simulink model "firmware"  (R2020a)
settings: Solver=FixedStepAuto  StartTime=0.0  StopTime=50.0  FixedStep=1e-3  RelTol=1e-3  EnableMultiTasking=on
undefined symbols (not defined in the file): A0, A1, A3, D0, D1, D10, D11, D12, D13, D2, D3, D4, D5, D6, D7, D8, D9, PTA0, PTA1, PTA2, PTB11, PTB2, PTB23, PTB3, PTB9, PTC16, PTC17, PTC2, PTC3, PTC4, PTD0, PTD1, PTD2, PTD3
libraries: etargetslib x44, frdmk64flib x22, dspstat3 x1
(part 2 of 2)

== system firmware/1.1.2 InputProcessing/1.1.2.4 CalculateUnsensedPace ==
  note: This block sets the LRL as a pulse period, later
      | used by AOO and VOO
  LowerRateLimit : Inport
  Data Type Conversion1 : DataTypeConversion  OutDataTypeStr=single
  Fcn2 : Fcn  Expr=u/60000
  Math Function1 : Math  Operator=reciprocal  SaturateOnIntegerOverflow=on
  f_aooInterval : Outport
  f_vooInterval : Outport  Port=2
  wires:
  Math Function1/1 -> f_vooInterval/1, f_aooInterval/1
  Data Type Conversion1/1 -> Fcn2/1
  Fcn2/1 -> Math Function1/1
  LowerRateLimit/1 -> Data Type Conversion1/1

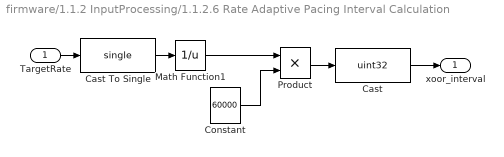
== system firmware/1.1.2 InputProcessing/1.1.2.6 Rate Adaptive Pacing Interval Calculation ==
  TargetRate : Inport  OutDataTypeStr=single
  Cast : DataTypeConversion  OutDataTypeStr=uint32
  Cast To Single : DataTypeConversion  OutDataTypeStr=single
  Constant : Constant  Value=60000
  Math Function1 : Math  Operator=reciprocal  SaturateOnIntegerOverflow=on
  Product : Product
  xoor_interval : Outport  OutDataTypeStr=uint32
  wires:
  Constant/1 -> Product/2
  Math Function1/1 -> Product/1
  Product/1 -> Cast/1
  Cast/1 -> xoor_interval/1
  TargetRate/1 -> Cast To Single/1
  Cast To Single/1 -> Math Function1/1

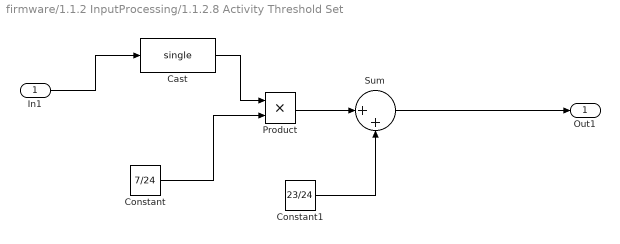
== system firmware/1.1.2 InputProcessing/1.1.2.8 Activity Threshold Set  ==
  In1 : Inport
  Cast : DataTypeConversion  OutDataTypeStr=single
  Constant : Constant  Value=7/24
  Constant1 : Constant  Value=23/24
  Product : Product
  Sum : Sum  Inputs=|++
  Out1 : Outport
  wires:
  Constant/1 -> Product/2
  Constant1/1 -> Sum/2
  Product/1 -> Sum/1
  Sum/1 -> Out1/1
  In1/1 -> Cast/1
  Cast/1 -> Product/1

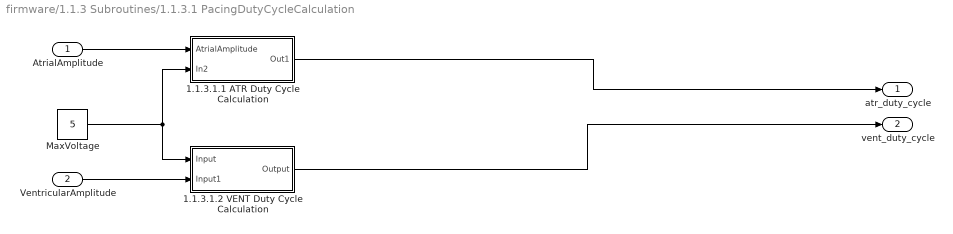
== system firmware/1.1.3 Subroutines/1.1.3.1 PacingDutyCycleCalculation ==
  AtrialAmplitude : Inport
  VentricularAmplitude : Inport  Port=2
  1.1.3.1.1 ATR Duty Cycle Calculation : Subsystem
  1.1.3.1.2 VENT Duty Cycle Calculation : Subsystem
  MaxVoltage : Constant  Value=5
  atr_duty_cycle : Outport
  vent_duty_cycle : Outport  Port=2
  wires:
  MaxVoltage/1 -> 1.1.3.1.2 VENT Duty Cycle Calculation/1(Input), 1.1.3.1.1 ATR Duty Cycle Calculation/2(In2)
  AtrialAmplitude/1 -> 1.1.3.1.1 ATR Duty Cycle Calculation/1(AtrialAmplitude)
  VentricularAmplitude/1 -> 1.1.3.1.2 VENT Duty Cycle Calculation/2(Input1)
  1.1.3.1.1 ATR Duty Cycle Calculation/1(Out1) -> atr_duty_cycle/1
  1.1.3.1.2 VENT Duty Cycle Calculation/1(Output) -> vent_duty_cycle/1

== system firmware/1.1.3 Subroutines/HIGH_or_LOW ==
  HIGH : Constant  Value=true
  LOW : Constant  Value=false
  Output : Outport
  Output1 : Outport  Port=2
  wires:
  LOW/1 -> Output1/1
  HIGH/1 -> Output/1

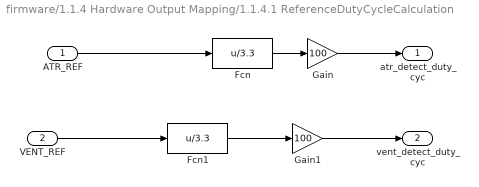
== system firmware/1.1.4 Hardware Output Mapping/1.1.4.1 ReferenceDutyCycleCalculation ==
  ATR_REF : Inport
  VENT_REF : Inport  Port=2
  Fcn : Fcn  Expr=u/3.3
  Fcn1 : Fcn  Expr=u/3.3
  Gain : Gain  Gain=100
  Gain1 : Gain  Gain=100
  atr_detect_duty_cyc : Outport
  vent_detect_duty_cyc : Outport  Port=2
  wires:
  Fcn/1 -> Gain/1
  VENT_REF/1 -> Fcn1/1
  Gain/1 -> atr_detect_duty_cyc/1
  Fcn1/1 -> Gain1/1
  Gain1/1 -> vent_detect_duty_cyc/1
  ATR_REF/1 -> Fcn/1

== system firmware/1.1.4 Hardware Output Mapping/1.1.4.2 Ventricular Pacing Inhibit ==
  VENT_CMP_REF_PWM : Inport
  VentPaceInhibit : Inport  Port=2
  Constant : Constant  Value=0
  Switch : Switch  Criteria=u2 > Threshold  Threshold=0.5
  Out1 : Outport
  wires:
  VENT_CMP_REF_PWM/1 -> Switch/3
  Constant/1 -> Switch/1
  VentPaceInhibit/1 -> Switch/2
  Switch/1 -> Out1/1

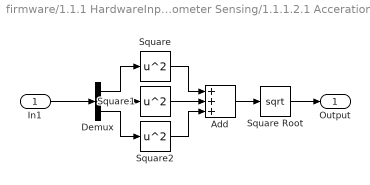
== system firmware/1.1.1 HardwareInputMapping/1.1.1.2 Accelerometer Sensing/1.1.1.2.1 Acceration Magnitude Calculation ==
  In1 : Inport
  Add : Sum  Inputs=+++
  Demux : Demux  Outputs=3
  Square : Math  Operator=square  SaturateOnIntegerOverflow=on
  Square Root : Sqrt  SaturateOnIntegerOverflow=on
  Square1 : Math  Operator=square  SaturateOnIntegerOverflow=on
  Square2 : Math  Operator=square  SaturateOnIntegerOverflow=on
  Output : Outport
  wires:
  Demux/1 -> Square/1
  Demux/2 -> Square1/1
  Demux/3 -> Square2/1
  Square/1 -> Add/1
  Square1/1 -> Add/2
  Square2/1 -> Add/3
  Add/1 -> Square Root/1
  Square Root/1 -> Output/1
  In1/1 -> Demux/1

== system firmware/1.1.3 Subroutines/1.1.3.1 PacingDutyCycleCalculation/1.1.3.1.1 ATR Duty Cycle Calculation ==
  AtrialAmplitude : Inport
  In2 : Inport  Port=2
  % : Constant  Value=100
  Divide : Product  Inputs=*/
  Product : Product
  Out1 : Outport
  wires:
  Divide/1 -> Product/1
  %/1 -> Product/2
  AtrialAmplitude/1 -> Divide/1
  In2/1 -> Divide/2
  Product/1 -> Out1/1

== system firmware/1.1.3 Subroutines/1.1.3.1 PacingDutyCycleCalculation/1.1.3.1.2 VENT Duty Cycle Calculation ==
  Input : Inport
  Input1 : Inport  Port=2
  % : Constant  Value=100
  Divide : Product  Inputs=*/
  Product : Product
  Output : Outport
  wires:
  Input/1 -> Divide/2
  Input1/1 -> Divide/1
  %/1 -> Product/2
  Divide/1 -> Product/1
  Product/1 -> Output/1

== stateflow chart firmware/1.1.2 InputProcessing/1.1.2.3 WatchdogTimerForPulseDetection ==
  state HysterisisSelection
    entry:
    time_minute = 60000; % ms/s
    smoothing_rate= InstHeartRate*(1-rs_down);
    total_lower_rate_time = 0;
  state DDDR
    entry:
    during:
    %tot_wait_time = time_minute-((ARP+AtrialPulseWidth)*smoothing_rate);
    %wait_time = tot_wait_time / smoothing_rate;
    total_XXIR_rate_time = time_minute-((p_v_a_r_p+AV_delay+AtrialPulseWidth)*XXIR_PPM);
    wait_time_XXIR= total_XXIR_rate_time/ XXIR_PPM;
    %For LRL so might not need for this mode, but again, left it here for now
    total_lower_rate_time = time_minute-((ARP+AtrialPulseWidth)*LRL);
    wait_time_LRL= total_lower_rate_time/ LRL;
    %For hysterisis so might not be needed for AAIR, but doesn't hurt to leave for now
    total_lower_rate_time_hys= time_minute - ((ARP + AtrialPulseWidth)*HRL);
    wait_time_LRL_hys= total_lower_rate_time_hys/ HRL;
  state AAI
    entry:
    tot_wait_time = time_minute-((ARP+AtrialPulseWidth)*smoothing_rate);
    wait_time = tot_wait_time / smoothing_rate;
    total_lower_rate_time = time_minute-((ARP+AtrialPulseWidth)*LRL);
    %total_lower_rate_time = time_minute - ((250 + 0.4)*50);
    wait_time_LRL= total_lower_rate_time/ LRL;
    %total_lower_rate_time_hys= time_minute - ((250 + 0.4)*45);
    %wait_time_LRL_hys= total_lower_rate_time_hys/ 45;
    total_lower_rate_time_hys= time_minute - ((ARP + AtrialPulseWidth)*HRL);
    wait_time_LRL_hys= total_lower_rate_time_hys/ HRL;
  state AAIR
    entry:
    during:
    %tot_wait_time = time_minute-((ARP+AtrialPulseWidth)*smoothing_rate);
    %wait_time = tot_wait_time / smoothing_rate;
    total_XXIR_rate_time = time_minute-((ARP+AtrialPulseWidth)*XXIR_PPM);
    wait_time_XXIR= total_XXIR_rate_time/ XXIR_PPM;
    %For LRL so might not need for this mode, but again, left it here for now
    total_lower_rate_time = time_minute-((ARP+AtrialPulseWidth)*LRL);
    wait_time_LRL= total_lower_rate_time/ LRL;
    %For hysterisis so might not be needed for AAIR, but doesn't hurt to leave for now
    total_lower_rate_time_hys= time_minute - ((ARP + AtrialPulseWidth)*HRL);
    wait_time_LRL_hys= total_lower_rate_time_hys/ HRL;
  state VVI
    entry:
    tot_wait_time = time_minute-((VRP+VentricularPulseWidth)*smoothing_rate);
    wait_time = tot_wait_time / smoothing_rate;
    %total_lower_rate_time = time_minute - ((320 + 1)*50);
    total_lower_rate_time = time_minute - ((VRP+VentricularPulseWidth)*LRL);
    wait_time_LRL= total_lower_rate_time/ LRL;
  state VVIR
    entry:
    during:
    %tot_wait_time = time_minute-((ARP+AtrialPulseWidth)*smoothing_rate);
    %wait_time = tot_wait_time / smoothing_rate;
    total_XXIR_rate_time = time_minute-((VRP+VentricularPulseWidth)*XXIR_PPM);
    wait_time_XXIR= total_XXIR_rate_time/ XXIR_PPM;
    %For LRL so might not need for this mode, but again, left it here for now
    total_lower_rate_time = time_minute-((VRP+VentricularPulseWidth)*LRL);
    wait_time_LRL= total_lower_rate_time/ LRL;
    %For hysterisis so might not be needed for AAIR, but doesn't hurt to leave for now
    total_lower_rate_time_hys= time_minute - ((VRP + VentricularPulseWidth)*HRL);
    wait_time_LRL_hys= total_lower_rate_time_hys/ HRL;
  (default) -> HysterisisSelection
  HysterisisSelection -> DDDR [order 2] : [Mode==3330]
  VVIR -> HysterisisSelection : [Mode ~= 2220]
  DDDR -> HysterisisSelection : [Mode ~=3330]
  HysterisisSelection -> VVIR [order 5] : [Mode == 2220]
  HysterisisSelection -> VVI [order 3] : [Mode==222]
  VVI -> HysterisisSelection : [Mode~=222]
  AAIR -> HysterisisSelection : [Mode ~=1120]
  HysterisisSelection -> AAI [order 1] : [Mode==112]
  HysterisisSelection -> AAIR [order 4] : [Mode==1120]
  AAI -> HysterisisSelection : [Mode ~= 112]
  data: HFlag input; Mode input; HRL input; LRL input uint32; AtrialPulseWidth input double; VentricularPulseWidth input double; InstHeartRate input double; VRP input uint32; rs_down input double; XXIR_PPM input; ARP input uint32; wait_time output; tot_wait_time local uint32; time_minute local uint32; smoothing_rate local double; wait_time_LRL output; total_lower_rate_time local uint32; wait_time_LRL_hys output; total_lower_rate_time_hys local; wait_time_XXIR output; total_XXIR_rate_time output uint32; p_v_a_r_p input; AV_delay input

== stateflow chart firmware/1.1.2 InputProcessing/1.1.2.7 AV Delay Determination ==
  state default
    entry:
  state fixed
    entry:
    AV_delay = fixed_AV
  state dynamic
    entry:
    AV_delay = min_AV + AV_offset + (1/current_HR)*5000
  (default) -> default
  default -> fixed [order 1] : [dyn_AV_delay ==  0]
  fixed -> default : [dyn_AV_delay ~= 0]
  dynamic -> default [order 1] : [dyn_AV_delay ~=1]
  default -> dynamic [order 2] : [dyn_AV_delay == 1]
  dynamic -> dynamic [order 2] : [after(1,msec)]
  data: fixed_AV input; min_AV input; AV_offset input; current_HR input; dyn_AV_delay input; AV_delay output single

== stateflow chart firmware/1.1.3 Subroutines/1.1.3.2 PacemakerControl ==
  state AOOR
    state CHARGE
      entry:
      ATR_PACE_CTRL=LOW;
      VENT_PACE_CTRL=LOW;
      PACING_REF_PWM=ATR_DUTY_CYCLE;
      PACE_CHARGE_CTRL=HIGH;
      PACE_GND_CTRL=HIGH;
      Z_ATR_CTRL=LOW;
      Z_VENT_CTRL=LOW;
      ATR_GND_CTRL=HIGH;
      VENT_GND_CTRL=LOW;
      %atrium_output_voltage = atrium_pulse_amplitude;
      %exit:
      %atrium_output_voltage = 0;
    state DISCHARGE
      entry:
      PACE_CHARGE_CTRL=LOW;
      PACE_GND_CTRL=HIGH;
      ATR_PACE_CTRL=HIGH;
      ATR_GND_CTRL=LOW;
      Z_ATR_CTRL=LOW;
      Z_VENT_CTRL=LOW;
      VENT_GND_CTRL=LOW;
      VENT_PACE_CTRL=LOW;
      PACING_REF_PWM=ATR_DUTY_CYCLE;
      %atrium_output_voltage = 0;
      %exit:
      %atrium_output_voltage = atrium_pulse_amplitude;
    (default) -> AOOR.CHARGE
    AOOR.DISCHARGE -> AOOR.CHARGE : [after(atrium_pulse_width,msec)]
    AOOR.CHARGE -> AOOR.DISCHARGE : [after(f_xoorInterval-atrium_pulse_width,msec)]
  state AAI
    state initializations
      entry:
      ATR_CMP_REF_PWM = ATR_SENS;
      %atrium_output_voltage  = 0;
      count=0;
    state Hysterisis_mode_ON
      entry:
      count = count +1;
    state Hysterisis_mode_OFF
      entry:
      count=count+1;
    state Pulse
      entry:
      %atrium_output_voltage = atrium_pulse_amplitude;
      ATR_PACE_CTRL=LOW;
      VENT_PACE_CTRL=LOW;
      PACING_REF_PWM=ATR_DUTY_CYCLE;
      PACE_CHARGE_CTRL=HIGH;
      PACE_GND_CTRL=HIGH;
      Z_ATR_CTRL=LOW;
      Z_VENT_CTRL=LOW;
      ATR_GND_CTRL=HIGH;
      VENT_GND_CTRL=LOW;
    state CHARGE
      entry:
      %atrium_output_voltage = atrium_pulse_amplitude;
      PACE_CHARGE_CTRL=LOW;
      PACE_GND_CTRL=HIGH;
      ATR_PACE_CTRL=HIGH;
      ATR_GND_CTRL=LOW;
      Z_ATR_CTRL=LOW;
      Z_VENT_CTRL=LOW;
      VENT_GND_CTRL=LOW;
      VENT_PACE_CTRL=LOW;
      PACING_REF_PWM=ATR_DUTY_CYCLE;
      %||((count>WaitTime) && (dig_atr_outputD0 == LOW))
    (default) -> AAI.initializations
    AAI.initializations -> AAI.Hysterisis_mode_ON [order 2] : [hysterisis_flag==1 && after(wait_time_LRL, msec)]
    AAI.initializations -> AAI.Hysterisis_mode_OFF [order 1] : [hysterisis_flag==0 && after(wait_time_LRL, msec)]
    AAI.Pulse -> AAI.initializations : [after(a_r_p,msec)]
    AAI.Hysterisis_mode_ON -> AAI.Hysterisis_mode_ON [order 2] : [(count<=WaitTime)&&(~(dig_atr_outputD0 == LOW && inst_heart_rate<lower_rate_limit))]
    AAI.Hysterisis_mode_OFF -> AAI.Hysterisis_mode_OFF [order 1] : [(count<=WaitTime)&&(~(dig_atr_outputD0 == LOW && inst_heart_rate<lower_rate_limit))]
    AAI.Hysterisis_mode_ON -> AAI.CHARGE [order 1] : [(dig_atr_outputD0 == LOW && inst_heart_rate<h_r_l)]
    AAI.Hysterisis_mode_OFF -> AAI.CHARGE [order 2] : [(dig_atr_outputD0 == LOW && inst_heart_rate<lower_rate_limit)]
    AAI.CHARGE -> AAI.Pulse : [after(atrium_pulse_width,msec)]
  state AAIR
    state initializations
      entry:
      ATR_CMP_REF_PWM = ATR_SENS;
      %atrium_output_voltage  = 0;
    state Hysterisis_mode_ON
      entry:
    state Hysterisis_mode_OFF
      entry:
    state Pulse
      entry:
      %atrium_output_voltage = atrium_pulse_amplitude;
      ATR_PACE_CTRL=LOW;
      VENT_PACE_CTRL=LOW;
      PACING_REF_PWM=ATR_DUTY_CYCLE;
      PACE_CHARGE_CTRL=HIGH;
      PACE_GND_CTRL=HIGH;
      Z_ATR_CTRL=LOW;
      Z_VENT_CTRL=LOW;
      ATR_GND_CTRL=HIGH;
      VENT_GND_CTRL=LOW;
    state CHARGE
      entry:
      %atrium_output_voltage = atrium_pulse_amplitude;
      PACE_CHARGE_CTRL=LOW;
      PACE_GND_CTRL=HIGH;
      ATR_PACE_CTRL=HIGH;
      ATR_GND_CTRL=LOW;
      Z_ATR_CTRL=LOW;
      Z_VENT_CTRL=LOW;
      VENT_GND_CTRL=LOW;
      VENT_PACE_CTRL=LOW;
      PACING_REF_PWM=ATR_DUTY_CYCLE;
      %||((count>WaitTime) && (dig_atr_outputD0 == LOW))
    (default) -> AAIR.initializations
    AAIR.initializations -> AAIR.Hysterisis_mode_ON [order 2] : [hysterisis_flag==1 && after(WaitTimeXXIR, msec)]
    AAIR.initializations -> AAIR.Hysterisis_mode_OFF [order 1] : [hysterisis_flag==0 && after(WaitTimeXXIR, msec)]
    AAIR.Pulse -> AAIR.initializations : [after(a_r_p,msec)]
    AAIR.Hysterisis_mode_ON -> AAIR.CHARGE : [(dig_atr_outputD0 == LOW  && inst_heart_rate<(CurrentRate-Hdiff))]
    AAIR.Hysterisis_mode_OFF -> AAIR.CHARGE : [(dig_atr_outputD0 == LOW  && inst_heart_rate<CurrentRate)]
    AAIR.CHARGE -> AAIR.Pulse : [after(atrium_pulse_width,msec)]
  state AOO
    state CHARGE
      entry:
      ATR_PACE_CTRL=LOW;
      VENT_PACE_CTRL=LOW;
      PACING_REF_PWM=ATR_DUTY_CYCLE;
      PACE_CHARGE_CTRL=HIGH;
      PACE_GND_CTRL=HIGH;
      Z_ATR_CTRL=LOW;
      Z_VENT_CTRL=LOW;
      ATR_GND_CTRL=HIGH;
      VENT_GND_CTRL=LOW;
      %atrium_output_voltage = atrium_pulse_amplitude;
      %exit:
      %atrium_output_voltage = 0;
    state DISCHARGE
      entry:
      PACE_CHARGE_CTRL=LOW;
      PACE_GND_CTRL=HIGH;
      ATR_PACE_CTRL=HIGH;
      ATR_GND_CTRL=LOW;
      Z_ATR_CTRL=LOW;
      Z_VENT_CTRL=LOW;
      VENT_GND_CTRL=LOW;
      VENT_PACE_CTRL=LOW;
      PACING_REF_PWM=ATR_DUTY_CYCLE;
      %atrium_output_voltage = 0;
      %exit:
      %atrium_output_voltage = atrium_pulse_amplitude;
    (default) -> AOO.CHARGE
    AOO.DISCHARGE -> AOO.CHARGE : [after(atrium_pulse_width,msec)]
    AOO.CHARGE -> AOO.DISCHARGE : [after(f_aooInterval-atrium_pulse_width,msec)]
  state Initialize
    entry:
    AOO = 100;
    VOO = 200;
    AAI = 112;
    VVI = 222;
    AOOR = 1000;
    AAIR = 1120;
    VOOR = 2000;
    VVIR = 2220;
    DDDR = 3330;
  state Standby
    entry:
    PACING_REF_PWM = 0;
  state DDDR
    state VENT_Pulse
      entry:
      ATR_PACE_CTRL=LOW;
      VENT_PACE_CTRL=LOW;
      PACING_REF_PWM=VENT_DUTY_CYCLE;
      PACE_CHARGE_CTRL=HIGH;
      PACE_GND_CTRL=HIGH;
      Z_ATR_CTRL=LOW;
      Z_VENT_CTRL=LOW;
      ATR_GND_CTRL=LOW;
      VENT_GND_CTRL=HIGH;
    state initializations
      entry:
      ATR_CMP_REF_PWM = ATR_SENS;
      VENT_CMP_REF_PWM = VENT_SENS;
    state VENT_CHARGE
      entry:
      PACE_CHARGE_CTRL=LOW;
      PACE_GND_CTRL=HIGH;
      ATR_PACE_CTRL=LOW;
      ATR_GND_CTRL=LOW;
      Z_ATR_CTRL=LOW;
      Z_VENT_CTRL=LOW;
      VENT_GND_CTRL=LOW;
      VENT_PACE_CTRL=HIGH;
      PACING_REF_PWM=VENT_DUTY_CYCLE;
    state Hysterisis_mode_ON
      entry:
    state Hysterisis_mode_OFF
      entry:
    state Sensing_Ventrical
      entry:
    state ATR_CHARGE
      entry:
      PACE_CHARGE_CTRL=LOW;
      PACE_GND_CTRL=HIGH;
      ATR_PACE_CTRL=HIGH;
      ATR_GND_CTRL=LOW;
      Z_ATR_CTRL=LOW;
      Z_VENT_CTRL=LOW;
      VENT_GND_CTRL=LOW;
      VENT_PACE_CTRL=LOW;
      PACING_REF_PWM=ATR_DUTY_CYCLE;
    state ATR_Pulse
      entry:
      ATR_PACE_CTRL=LOW;
      VENT_PACE_CTRL=LOW;
      PACING_REF_PWM=ATR_DUTY_CYCLE;
      PACE_CHARGE_CTRL=HIGH;
      PACE_GND_CTRL=HIGH;
      Z_ATR_CTRL=LOW;
      Z_VENT_CTRL=LOW;
      ATR_GND_CTRL=HIGH;
      VENT_GND_CTRL=LOW;
    (default) -> DDDR.initializations
    DDDR.initializations -> DDDR.Hysterisis_mode_ON [order 2] : [hysterisis_flag==1 && after(WaitTimeXXIR, msec)]
    VENT_Pulse -> DDDR.initializations : [after(p_v_a_r_p,msec)]
    DDDR.initializations -> DDDR.Hysterisis_mode_OFF [order 1] : [hysterisis_flag==0 && after(WaitTimeXXIR, msec)]
    ATR_Pulse -> DDDR.initializations [order 2] : [dig_vent_outputD1 == HIGH]
    Sensing_Ventrical -> DDDR.initializations [order 1] : [dig_vent_outputD1 == HIGH]
    DDDR.initializations -> Sensing_Ventrical [order 3] : [dig_atr_outputD0 == HIGH]
    VENT_CHARGE -> VENT_Pulse : [after(ventricle_pulse_width,msec)]
    DDDR.Hysterisis_mode_ON -> Sensing_Ventrical [order 2] : [dig_atr_outputD0 == HIGH && inst_heart_rate<(CurrentRate-Hdiff)]
    DDDR.Hysterisis_mode_OFF -> Sensing_Ventrical [order 2] : [dig_atr_outputD0 == HIGH && inst_heart_rate<CurrentRate]
    DDDR.Hysterisis_mode_OFF -> ATR_CHARGE [order 1] : [(dig_atr_outputD0 == LOW  && inst_heart_rate<CurrentRate)]
    DDDR.Hysterisis_mode_ON -> ATR_CHARGE [order 1] : [(dig_atr_outputD0 == LOW  && inst_heart_rate<(CurrentRate-Hdiff))]
    Sensing_Ventrical -> VENT_CHARGE [order 2] : [after(AV_delay-1,msec)]
    ATR_Pulse -> Sensing_Ventrical [order 1] : [after(1,msec)]
    ATR_CHARGE -> ATR_Pulse : [after(atrium_pulse_width,msec)]
  state VVI
    state initializations
      entry:
      VENT_CMP_REF_PWM = VENT_SENS;
      %ventricle_output_voltage  = 0;
      count=0;
    state Hysterisis_mode_OFF
      entry:
      count=count+1
    state Pulse
      entry:
      %ventricle_output_voltage = ventricle_pulse_amplitude;
      ATR_PACE_CTRL=LOW;
      VENT_PACE_CTRL=LOW;
      PACING_REF_PWM=VENT_DUTY_CYCLE;
      PACE_CHARGE_CTRL=HIGH;
      PACE_GND_CTRL=HIGH;
      Z_ATR_CTRL=LOW;
      Z_VENT_CTRL=LOW;
      ATR_GND_CTRL=LOW;
      VENT_GND_CTRL=HIGH;
    state Hysterisis_mode_ON
      entry:
      count = count +1;
    state CHARGE
      entry:
      %ventricle_output_voltage = ventricle_pulse_amplitude;
      PACE_CHARGE_CTRL=LOW;
      PACE_GND_CTRL=HIGH;
      ATR_PACE_CTRL=LOW;
      ATR_GND_CTRL=LOW;
      Z_ATR_CTRL=LOW;
      Z_VENT_CTRL=LOW;
      VENT_GND_CTRL=LOW;
      VENT_PACE_CTRL=HIGH;
      PACING_REF_PWM=VENT_DUTY_CYCLE;
      %||((count>WaitTime) && (dig_vent_outputD1 == LOW))
    (default) -> VVI.initializations
    VVI.initializations -> VVI.Hysterisis_mode_ON [order 2] : [hysterisis_flag==1 && after(wait_time_LRL, msec)]
    VVI.initializations -> VVI.Hysterisis_mode_OFF [order 1] : [hysterisis_flag==0 && after(wait_time_LRL, msec)]
    VVI.Pulse -> VVI.initializations : [after(v_r_p,msec)]
    VVI.Hysterisis_mode_OFF -> VVI.Hysterisis_mode_OFF [order 1] : [(count<=WaitTime)&&(~(dig_vent_outputD1 == LOW && inst_heart_rate<lower_rate_limit))]
    VVI.Hysterisis_mode_ON -> VVI.Hysterisis_mode_ON [order 2] : [(count<=WaitTime)&&(~(dig_vent_outputD1 == LOW && inst_heart_rate<lower_rate_limit))]
    VVI.Hysterisis_mode_OFF -> VVI.CHARGE [order 2] : [(dig_vent_outputD1 == LOW && inst_heart_rate<lower_rate_limit)]
    VVI.Hysterisis_mode_ON -> VVI.CHARGE [order 1] : [(dig_vent_outputD1 == LOW && inst_heart_rate<h_r_l)]
    VVI.CHARGE -> VVI.Pulse : [after(ventricle_pulse_width,msec)]
  state VOO
    state CHARGE
      entry:
      ATR_PACE_CTRL=LOW;
      VENT_PACE_CTRL=LOW;
      PACING_REF_PWM=VENT_DUTY_CYCLE;
      PACE_CHARGE_CTRL=HIGH;
      PACE_GND_CTRL=HIGH;
      Z_ATR_CTRL=LOW;
      Z_VENT_CTRL=LOW;
      ATR_GND_CTRL=LOW;
      VENT_GND_CTRL=HIGH;
      %atrium_output_voltage = atrium_pulse_amplitude;
      %exit:
      %atrium_output_voltage = 0;
    state DISCHARGE
      entry:
      PACE_CHARGE_CTRL=LOW;
      PACE_GND_CTRL=HIGH;
      ATR_PACE_CTRL=LOW;
      ATR_GND_CTRL=LOW;
      Z_ATR_CTRL=LOW;
      Z_VENT_CTRL=LOW;
      VENT_GND_CTRL=LOW;
      VENT_PACE_CTRL=HIGH;
      PACING_REF_PWM=VENT_DUTY_CYCLE;
      %ventricle_output_voltage = 0;
      %exit:
      %ventricle_output_voltage = ventricle_pulse_amplitude;
    (default) -> VOO.CHARGE
    VOO.DISCHARGE -> VOO.CHARGE : [after(ventricle_pulse_width,msec)]
    VOO.CHARGE -> VOO.DISCHARGE : [after(f_vooInterval-ventricle_pulse_width,msec)]
  state VVIR
    state initializations
      entry:
      VENT_CMP_REF_PWM = VENT_SENS;
    state Hysterisis_mode_ON
      entry:
    state Hysterisis_mode_OFF
      entry:
    state Pulse
      entry:
      %atrium_output_voltage = atrium_pulse_amplitude;
      ATR_PACE_CTRL=LOW;
      VENT_PACE_CTRL=LOW;
      PACING_REF_PWM=VENT_DUTY_CYCLE;
      PACE_CHARGE_CTRL=HIGH;
      PACE_GND_CTRL=HIGH;
      Z_ATR_CTRL=LOW;
      Z_VENT_CTRL=LOW;
      ATR_GND_CTRL=LOW;
      VENT_GND_CTRL=HIGH;
    state CHARGE
      entry:
      %atrium_output_voltage = atrium_pulse_amplitude;
      PACE_CHARGE_CTRL=LOW;
      PACE_GND_CTRL=HIGH;
      ATR_PACE_CTRL=LOW;
      ATR_GND_CTRL=LOW;
      Z_ATR_CTRL=LOW;
      Z_VENT_CTRL=LOW;
      VENT_GND_CTRL=LOW;
      VENT_PACE_CTRL=HIGH;
      PACING_REF_PWM=VENT_DUTY_CYCLE;
    (default) -> VVIR.initializations
    VVIR.initializations -> VVIR.Hysterisis_mode_ON [order 2] : [hysterisis_flag==1 && after(WaitTimeXXIR, msec)]
    VVIR.initializations -> VVIR.Hysterisis_mode_OFF [order 1] : [hysterisis_flag==0 && after(WaitTimeXXIR, msec)]
    VVIR.Pulse -> VVIR.initializations : [after(v_r_p,msec)]
    VVIR.Hysterisis_mode_ON -> VVIR.CHARGE : [(dig_vent_outputD1 == LOW  && inst_heart_rate<(CurrentRate-Hdiff))]
    VVIR.Hysterisis_mode_OFF -> VVIR.CHARGE : [(dig_vent_outputD1 == LOW  && inst_heart_rate<CurrentRate)]
    VVIR.CHARGE -> VVIR.Pulse : [after(ventricle_pulse_width,msec)]
  state VOOR
    state CHARGE
      entry:
      ATR_PACE_CTRL=LOW;
      VENT_PACE_CTRL=LOW;
      PACING_REF_PWM=VENT_DUTY_CYCLE;
      PACE_CHARGE_CTRL=HIGH;
      PACE_GND_CTRL=HIGH;
      Z_ATR_CTRL=LOW;
      Z_VENT_CTRL=LOW;
      ATR_GND_CTRL=LOW;
      VENT_GND_CTRL=HIGH;
      %atrium_output_voltage = atrium_pulse_amplitude;
      %exit:
      %atrium_output_voltage = 0;
    state DISCHARGE
      entry:
      PACE_CHARGE_CTRL=LOW;
      PACE_GND_CTRL=HIGH;
      ATR_PACE_CTRL=LOW;
      ATR_GND_CTRL=LOW;
      Z_ATR_CTRL=LOW;
      Z_VENT_CTRL=LOW;
      VENT_GND_CTRL=LOW;
      VENT_PACE_CTRL=HIGH;
      PACING_REF_PWM=VENT_DUTY_CYCLE;
      %ventricle_output_voltage = 0;
      %exit:
      %ventricle_output_voltage = ventricle_pulse_amplitude;
    (default) -> VOOR.CHARGE
    VOOR.DISCHARGE -> VOOR.CHARGE : [after(ventricle_pulse_width,msec)]
    VOOR.CHARGE -> VOOR.DISCHARGE : [after(f_xoorInterval-ventricle_pulse_width,msec)]
  AOOR -> Standby : [mode ~= AOOR]
  Standby -> AOOR [order 2] : [mode == AOOR]
  AOO -> Standby : [mode ~= AOO]
  Standby -> AOO [order 1] : [mode == AOO]
  AAI -> Standby : [mode ~= AAI]
  Standby -> AAI [order 8] : [mode == AAI]
  AAIR -> Standby : [mode ~= AAIR]
  Standby -> AAIR [order 5] : [mode == AAIR]
  (default) -> Initialize
  Standby -> DDDR [order 10] : [mode == DDDR]
  Initialize -> Standby : [HR_Ready == true]
  DDDR -> Standby : [mode ~= DDDR]
  Standby -> Initialize [order 9] : [HR_Ready == false]
  VOO -> Standby : [mode ~= VOO]
  Standby -> VOO [order 7] : [mode == VOO]
  VOOR -> Standby : [mode ~= VOOR]
  Standby -> VOOR [order 4] : [mode == VOOR]
  VVIR -> Standby : [mode ~= VVIR]
  Standby -> VVIR [order 3] : [mode == VVIR]
  VVI -> Standby : [mode ~= VVI]
  Standby -> VVI [order 6] : [mode == VVI]
  data: mode input uint32; upper_rate_limit input uint32; lower_rate_limit input uint32; atrium_pulse_width input double; ventricle_pulse_width input double; f_aooInterval input single; f_vooInterval input single; AAI local uint32; VVI local uint32; VOO local int32; AOO local uint32; WaitTime input; dig_vent_outputD1 input; avg_heart_rate input; inst_heart_rate input; dig_atr_outputD0 input; hysterisis_flag input; v_r_p input; a_r_p input; prev_inst_heart_rate input; h_r_l input; ATR_GND_CTRL output; ATR_PACE_CTRL output; PACE_CHARGE_CTRL output; PACE_GND_CTRL output; PACING_REF_PWM output; VENT_GND_CTRL output; VENT_PACE_CTRL output; Z_ATR_CTRL output; Z_VENT_CTRL output; HIGH input; LOW input; ATR_DUTY_CYCLE input; VENT_DUTY_CYCLE input; ATR_CMP_REF_PWM output; VENT_CMP_REF_PWM output; VENT_SENS input; ATR_SENS input; HR_Ready input boolean; count output; p_v_a_r_p input; wait_time_hys input; wait_time_LRL input; activity_index input; Recovery_Time input; MSRate input; Reaction_Time input; RF input; f_xoorInterval input; AOOR local; VVIR local; VOOR local; AAIR local; VLOW local; VHIGH local; MHIGH local; MED local; LLOW local; HHIGH local; ActivityThreshold input; XXIR_PPM input; WaitTimeXXIR input; CurrentRate input; DDDR local; AV_delay input; Hdiff input; atrium_output_voltage local single; ventricle_output_voltage local single

== stateflow chart firmware/1.1.2 InputProcessing/1.1.2.1 PulsePeriodDetermination ==
  state default
    entry:
  state UnsensedModes
    entry:
    HR_Ready = true
    exit:
    HR_Ready = false
  state AtrialRateDetection
    state default
      entry:
      pulse_finished = false
      time_between_pulses = 0
    state setARPasDeltaT
      entry:
      time_between_pulses = ARP
    state awaitNewPulse
      entry:
      time_between_pulses = time_between_pulses+1
    state newPulseDetected
      entry:
      pulse_finished = true
      HR_Ready = true
    state resetDeltaT
      entry:
      pulse_finished = false
      time_between_pulses = ARP
    (default) -> AtrialRateDetection.default
    AtrialRateDetection.default -> setARPasDeltaT : [AtrialPulseDetected == 1]
    setARPasDeltaT -> (junction 59) : [after(ARP,msec)]
    AtrialRateDetection.awaitNewPulse -> AtrialRateDetection.awaitNewPulse [order 1] : [AtrialPulseDetected == 0]
    (junction 59) -> AtrialRateDetection.awaitNewPulse [order 1] : [AtrialPulseDetected ==0]
    (junction 59) -> AtrialRateDetection.newPulseDetected [order 2] : [AtrialPulseDetected == 1]
    AtrialRateDetection.resetDeltaT -> (junction 59) : [after(ARP-1,msec)]
    AtrialRateDetection.awaitNewPulse -> AtrialRateDetection.newPulseDetected [order 2] : [AtrialPulseDetected == 1]
    AtrialRateDetection.newPulseDetected -> AtrialRateDetection.resetDeltaT : [after(1,msec)]
  state VenticularRateDetection
    state default
      entry:
      pulse_finished = false
      time_between_pulses = 0
    state setVRPasDeltaT
      entry:
      time_between_pulses = VRP
    state awaitNewPulse
      entry:
      time_between_pulses = time_between_pulses+1
    state newPulseDetected
      entry:
      pulse_finished = true
      HR_Ready = true
    state resetDeltaT
      entry:
      pulse_finished = false
      time_between_pulses = VRP
    (default) -> VenticularRateDetection.default
    VenticularRateDetection.default -> setVRPasDeltaT : [VentricularPulseDetected == 1]
    setVRPasDeltaT -> (junction 93) : [after(VRP,msec)]
    VenticularRateDetection.awaitNewPulse -> VenticularRateDetection.awaitNewPulse [order 1] : [VentricularPulseDetected == 0]
    (junction 93) -> VenticularRateDetection.awaitNewPulse [order 1] : [VentricularPulseDetected ==0]
    (junction 93) -> VenticularRateDetection.newPulseDetected [order 2] : [VentricularPulseDetected == 1]
    VenticularRateDetection.resetDeltaT -> (junction 93) : [after(VRP-1,msec)]
    VenticularRateDetection.awaitNewPulse -> VenticularRateDetection.newPulseDetected [order 2] : [VentricularPulseDetected == 1]
    VenticularRateDetection.newPulseDetected -> VenticularRateDetection.resetDeltaT : [after(1,msec)]
  (default) -> default
  default -> UnsensedModes [order 2] : [Mode == 100 || Mode == 200]
  UnsensedModes -> default : [Mode ~= 100 && Mode ~= 200]
  default -> AtrialRateDetection [order 1] : [Mode == 112 || Mode == 1120 || Mode == 3330]
  AtrialRateDetection -> default : [Mode ~= 112 && Mode ~= 1120 && Mode ~= 3330]
  default -> VenticularRateDetection [order 3] : [Mode == 222 || Mode == 2220]
  VenticularRateDetection -> default : [Mode ~= 222 && Mode ~= 2220]
  data: Mode input; time_between_pulses output uint32; pulse_finished output boolean; AtrialPulseDetected input boolean; VentricularPulseDetected input boolean; VRP input uint32; ARP input uint32; HR_Ready output boolean

== stateflow chart firmware/1.1.1 HardwareInputMapping/1.1.1.1 Accelerometer Trigger ==
  state default
    entry:
    trigger = false
  state accelerometer_on
    entry:
    trigger = true
  (default) -> default
  default -> accelerometer_on : [after(50,msec)]
  accelerometer_on -> default : [after(50,msec)]
  data: trigger output boolean

== stateflow chart firmware/1.1.1 HardwareInputMapping/1.1.1.3 Recieved Serial Message Processing ==
  state Write_Data
    entry:
    % Set new values for parameters
    % --- uint32 values = values - 1-
    Mode                   = Mode_U;
    upper_rate_limit       = upper_rate_limit_U;
    lower_rate_limit       = lower_rate_limit_U;
    a_r_p                  = a_r_p_U;
    p_v_a_r_p              = p_v_a_r_p_U;
    h_r_l                  = h_r_l_U;
    v_r_p                  = v_r_p_U;
    activity_threshold     = activity_threshold_U;
    ReactionTime           = ReactionTime_U;
    ResponseFactor         = ResponseFactor_U;
    RecoveryTime           = RecoveryTime_U;
    MSR                    = MSR_U;
    Fixed_AV_delay         = Fixed_AV_delay_U;
    p_v_a_r_p_ext          = p_v_a_r_p_ext_U;
    ATR_dur                = ATR_dur_U;
    % --- uint8 values = values - 1-
    hysterisis_flag        = hysterisis_flag_U;
    Dynamic_AV_delay       = Dynamic_AV_delay_U;
    ATR_fallback_time      = ATR_fallback_time_U;
    ATR_mode               = ATR_mode_U;
    vent_blanking          = vent_blanking_U;
    min_AV_delay           = min_AV_delay_U;
    % --- int8 value = value - 1-
    sensed_AV_delay_offset = sensed_AV_delay_offset_U;
    % --- single (float32) values = values - 1-
    atrial_amplitude          = atrial_amplitude_U;
    ventricular_amplitude     = ventricular_amplitude_U;
    atrial_sensitivity        = atrial_sensitivity_U;
    ventricular_sensitivity   = ventricular_sensitivity_U;
    atrial_amplitude_Re       = atrial_amplitude_Re_U;
    ventricular_amplitude_Re  = ventricular_amplitude_Re_U;
    % --- double (float64) values = values - 1-
    atrial_pulse_width        = atrial_pulse_width_U;
    ventricular_pulse_width   = ventricular_pulse_width_U;
    r_s_up                    = r_s_up_U;
    r_s_down                  = r_s_down_U;
    % --- Manual overrides
    ventricular_sensitivity = 2.5;
    atrial_sensitivity      = 2.75;
  state Echo
    entry:
    MSG_trigger = 1;
    MSG_ident = 2;
  state UpdateFailed
    % Set default values for parameters
    entry:
  state Safety_Check
    entry:
    safety_flag = true;
    while(safety_flag == true)
    if  (~(50<=upper_rate_limit_U<=175))
    safety_flag = false;
    end
    if  (~(50<=lower_rate_limit_U<=upper_rate_limit))
    safety_flag = false;
    end
    if (Mode_U ~= 100 && Mode_U ~= 200 && Mode_U ~= 112 && Mode_U ~= 222 && Mode_U ~= 1000 && Mode_U ~= 1120 && Mode_U ~= 2000 && Mode_U ~= 2220 && Mode_U ~= 3330)
    safety_flag = false;
    end
    break
    end
  state par_load
    entry:
    MSG_trigger = 1;
    MSG_ident = 3;
  state Initial_State
    % Set default values for parameters
    entry:
    Mode = 100;
    upper_rate_limit = 175;
    lower_rate_limit = 60;
    atrial_amplitude = 3.75;
    atrial_pulse_width = 0.4;
    ventricular_amplitude = 3.75;
    ventricular_pulse_width = 1;
    a_r_p = 250;
    p_v_a_r_p = 250;
    h_r_l = 45;
    r_s_up = 0.09;
    r_s_down = 0.09;
    ventricular_sensitivity = 2.5;
    atrial_sensitivity = 2.75
    v_r_p = 320;
    hysterisis_flag = 0; % should talk about it
    activity_threshold = 2;
    ReactionTime = 10;
    ResponseFactor = 6;
    RecoveryTime = 2;
    MSR = 120;
  state Read_Data
    entry:
    % --- uint32 (4 bytes) ---
    tmp_u32 = typecast(uint8(rx_data(3:6)), 'uint32'); Mode_U = tmp_u32(1);
    tmp_u32 = typecast(uint8(rx_data(7:10)), 'uint32');   upper_rate_limit_U = tmp_u32(1);
    tmp_u32 = typecast(uint8(rx_data(11:14)), 'uint32');  lower_rate_limit_U = tmp_u32(1);
    tmp_u32 = typecast(uint8(rx_data(39:42)), 'uint32');  a_r_p_U = tmp_u32(1);
    tmp_u32 = typecast(uint8(rx_data(43:46)), 'uint32');  p_v_a_r_p_U = tmp_u32(1);
    tmp_u32 = typecast(uint8(rx_data(47:50)), 'uint32');  h_r_l_U = tmp_u32(1);
    tmp_u32 = typecast(uint8(rx_data(75:78)), 'uint32');  v_r_p_U = tmp_u32(1);
    tmp_u32 = typecast(uint8(rx_data(79:82)), 'uint32');  activity_threshold_U = tmp_u32(1);
    tmp_u32 = typecast(uint8(rx_data(83:86)), 'uint32');  ReactionTime_U = tmp_u32(1);
    tmp_u32 = typecast(uint8(rx_data(87:90)), 'uint32');  ResponseFactor_U = tmp_u32(1);
    tmp_u32 = typecast(uint8(rx_data(91:94)), 'uint32');  RecoveryTime_U = tmp_u32(1);
    tmp_u32 = typecast(uint8(rx_data(95:98)), 'uint32');  MSR_U = tmp_u32(1);
    tmp_u32 = typecast(uint8(rx_data(108:111)), 'uint32'); Fixed_AV_delay_U = tmp_u32(1);
    tmp_u32 = typecast(uint8(rx_data(114:117)), 'uint32'); p_v_a_r_p_ext_U = tmp_u32(1);
    tmp_u32 = typecast(uint8(rx_data(118:121)), 'uint32'); ATR_dur_U = tmp_u32(1);
    % --- uint8 (1 byte) ---
    hysterisis_flag_U = uint8(rx_data(99));
    Dynamic_AV_delay_U = uint8(rx_data(112));
    ATR_fallback_time_U =  uint8(rx_data(122));
    ATR_mode_U =  uint8(rx_data(123));
    vent_blanking_U =  uint8(rx_data(124));
    min_AV_delay_U =  uint8(rx_data(125));
    % --- int8 (1 byte) ---
    sensed_AV_delay_offset_U = int8(rx_data(113));
    % --- single (float32, 4 bytes) ---
    tmp_single = typecast(uint8(rx_data(15:18)), 'single');  atrial_amplitude_U = tmp_single(1);
    tmp_single = typecast(uint8(rx_data(27:30)), 'single');  ventricular_amplitude_U = tmp_single(1);
    tmp_single = typecast(uint8(rx_data(67:70)), 'single');  atrial_sensitivity_U = tmp_single(1);
    tmp_single = typecast(uint8(rx_data(71:74)), 'single');  ventricular_sensitivity_U = tmp_single(1);
    tmp_single = typecast(uint8(rx_data(100:103)),'single'); atrial_amplitude_Re_U = tmp_single(1);
    tmp_single = typecast(uint8(rx_data(104:107)),'single'); ventricular_amplitude_Re_U = tmp_single(1);
    % --- double (float64, 8 bytes) ---
    tmp_double = typecast(uint8(rx_data(19:26)), 'double');  atrial_pulse_width_U = tmp_double(1);
    tmp_double = typecast(uint8(rx_data(31:38)), 'double');  ventricular_pulse_width_U = tmp_double(1);
    tmp_double = typecast(uint8(rx_data(51:58)), 'double');  r_s_up_U = tmp_double(1);
    tmp_double = typecast(uint8(rx_data(59:66)), 'double');  r_s_down_U = tmp_double(1);
  state Standby
    entry:
    MSG_trigger = 0;
  state HandshakeRequestEnable
    entry:
    MSG_trigger = 1;
    MSG_ident = 1;
  state Egram_Update
    entry:
    MSG_trigger =1;
    MSG_ident =0;
  Safety_Check -> Write_Data [order 2] : [safety_flag == true]
  Write_Data -> Echo
  Echo -> (junction 81)
  UpdateFailed -> Echo
  Safety_Check -> UpdateFailed [order 1] : [safety_flag == false]
  (junction 81) -> Standby
  (default) -> Initial_State
  par_load -> Standby
  (junction 12) -> par_load [order 4] : [[[rx_data(2) == hex2dec('60')]]]
  Initial_State -> Standby
  Standby -> (junction 7) : [status==0]
  (junction 12) -> Read_Data [order 1] : [[rx_data(2) == hex2dec('55')]]
  (junction 7) -> (junction 12) : [[rx_data(1) == hex2dec('16')]]
  (junction 12) -> HandshakeRequestEnable [order 2] : [[[rx_data(2) == hex2dec('45')]]]
  (junction 12) -> Egram_Update [order 3] : [[rx_data(2) == hex2dec('36')]]
  Egram_Update -> Standby
  HandshakeRequestEnable -> Standby : [after(1,msec)]
  Read_Data -> Safety_Check : [after(1,msec)]
  data: MSG_ident output uint8; rx_data input; MSR output uint32; ReactionTime output uint32; Mode output uint32; RecoveryTime output uint32; ResponseFactor output uint32; a_r_p output uint32; activity_threshold output uint32; atrial_amplitude output single; atrial_pulse_width output; atrial_sensitivity output single; h_r_l output uint32; hysterisis_flag output uint8; lower_rate_limit output uint32; p_v_a_r_p output uint32; r_s_down output; r_s_up output; upper_rate_limit output uint32; v_r_p output uint32; ventricular_amplitude output single; ventricular_pulse_width output; ventricular_sensitivity output single; MSR_U local uint32; Mode_U local; ReactionTime_U local; RecoveryTime_U local; ResponseFactor_U local; a_r_p_U local; activity_threshold_U local; atrial_amplitude_U local; atrial_pulse_width_U local; atrial_sensitivity_U local; h_r_l_U local; hysterisis_flag_U local; lower_rate_limit_U local; p_v_a_r_p_U local; r_s_down_U local; r_s_up_U local; upper_rate_limit_U local; v_r_p_U local; ventricular_amplitude_U local; ventricular_pulse_width_U local; ventricular_sensitivity_U local; tmp_double local size=8 [1..8]; tmp_u32 local size=8 [1..12]; tmp_single local size=4 [1..4]; status input size=1; safety_flag local boolean; MSG_trigger output uint8; ATR_dur_U local uint32; ATR_fallback_time_U local uint8; ATR_mode_U local uint8; Dynamic_AV_delay_U local uint8; Fixed_AV_delay_U local uint32; atrial_amplitude_Re_U local single; ventricular_amplitude_Re_U local single; min_AV_delay_U local uint8; p_v_a_r_p_ext_U local uint32; sensed_AV_delay_offset_U local int8; vent_blanking_U local uint8; ATR_dur output uint32; ATR_fallback_time output uint8; ATR_mode output uint8; Dynamic_AV_delay output uint8; Fixed_AV_delay output uint32; atrial_amplitude_Re output single; ventricular_amplitude_Re output single; min_AV_delay output uint8; p_v_a_r_p_ext output uint32; sensed_AV_delay_offset output int8; vent_blanking output uint8

== stateflow chart firmware/1.1.2 InputProcessing/1.1.2.5 Rate Adaptive Pacing Calculation ==
  state start
    entry:
    DesiredRate = LowerRateLimit;
    CR = LowerRateLimit;
  state default
    entry:
    LED_flag=0;
    during:
    DesiredRate = LowerRateLimit;
    CR = LowerRateLimit;
    stepup=((MSR-LowerRateLimit)/ReactionTime);
    stepdown=((MSR-LowerRateLimit)/(RecoveryTime*60));
    Local_Mode = Mode;
  state stepdown
    entry:
    CR=CR-stepdown;
    LED_flag = 0;
  state overThreshold
    entry:
    LED_flag = 1;
    CR = DesiredRate;
    %DesiredRate = MSR;
    during:
    DesiredRate = LowerRateLimit + (MSR-LowerRateLimit)*(1-2.718^(-1*ResponseFactor*((4*activity_magnitude) - ActivityThreshold)));
  state STEPUP
    entry:
    CR=CR+stepup;
  (default) -> start
  start -> default
  stepdown -> default [order 3] : [Local_Mode ~= Mode]
  STEPUP -> default [order 3] : [Local_Mode ~= Mode]
  stepdown -> default [order 2] : [CR <= LowerRateLimit]
  default -> overThreshold : [activity_magnitude >= ActivityThreshold]
  stepdown -> stepdown [order 1] : [after(1,sec)]
  overThreshold -> stepdown [order 1] : [activity_magnitude < ActivityThreshold]
  overThreshold -> STEPUP [order 2] : [CR<DesiredRate]
  STEPUP -> overThreshold [order 2] : [CR >= DesiredRate]
  STEPUP -> STEPUP [order 1] : [after(1,sec)]
  data: RecoveryTime input; ReactionTime input; activity_magnitude input single; MSR input single; LowerRateLimit input single; ResponseFactor input single; ActivityThreshold input single; LED_flag output uint32; DesiredRate output single; CR output; stepdown local single; Mode input; Local_Mode local; stepup local single
